simulink library "commdigbbndcpm2"  (Simulink 6.0)
settings: Solver=ode45  SolverMode=SingleTasking  StartTime=0.0  StopTime=10.0  RelTol=1e-3
libraries: commdigbbndcpm2 x6
settings Model: RequirementInfo=9  Creator=tdelve  LastModifiedBy=cvora  ExtModeAutoUpdateStatusClock=off  ProdHWDeviceType=Specified
settings DataIOCC: SignalLoggingName=logsOut
settings OptimizationCC: BooleanDataType=off
settings DebuggingCC: CheckExecutionContextPreStartOutputMsg=on  CheckExecutionContextRuntimeOutputMsg=on  SolverPrmCheckMsg=none
settings HardwareCC: ProdHWDeviceType=Specified
settings SFSimCC: SFSimApplyToAllLibs=on  SFSimBuildMode=Incremental

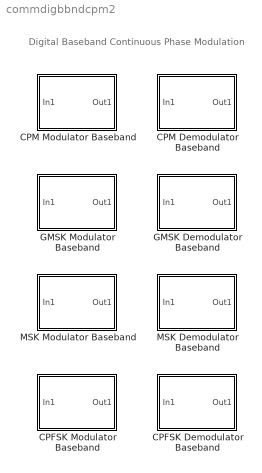
== system commdigbbndcpm2 ==
  note: Digital Baseband
      | Continuous Phase Modulation
  CPFSK Demodulator Baseband : Subsystem  PropExecContextAcrossSSBoundary=on  mask(CPFSK Demodulator Baseband){Mnum=4, outputType=Integer, mappingType=Binary, modIdx=.5, phaseOffset=0, samplesPerSymbol=8, traceBack=16}
      mask prompts: Mnum "M-ary number:"; outputType "Output type:"; mappingType "Symbol set ordering:"; modIdx "Modulation index:"; phaseOffset "Phase offset (rad):"; samplesPerSymbol "Samples per symbol:"; traceBack "Traceback length:"
      mask help:
      | Demodulate the CPFSK modulated input signal using the Viterbi algorithm. Traceback length is the number of trellis branches that the algorithm uses to construct each traceback path.
      |
      | For sample-based input, the input must be a scalar. For frame-based input, the input must be a column vector.
      |
      | The output can be either bits or integers. In case of bit output, the output width is an integer multiple of the number of bits per symbol. The symbols can be either binary-demapped or Gray-demapped into bits.
      |
      | In case of frame-based input, the width of the input frame represents the product of the number of symbols and the Samples per symbol value.
      |
      | In case of sample-based input, the sample time of the input is the symbol period divided by the Samples per symbol value.
      mask init:
      | [eStr,params]=commblkcpfskdemod(gcb, 'init');
      | if(eStr.ecode==1)
      |     error(eStr.emsg);
      | elseif(eStr.ecode==2)
      |     warning(eStr.emsg);
      | end;
      settings: ErrorFcn=commblkcpfskdemod
      mask Help: helpview(commbhelp)
      mask StyleString: edit,popup(Bit|Integer),popup(Binary|Gray),edit,edit,edit,edit
      mask CallbackString: |commblkcpfskdemod(gcb,'cbOutputType');|||||
      mask Display:
      | plot(0,0,100,100,[5+1.5*[[0:.8:10] [10:1.6:20] [20:.8:30]] 50 50 50 50+15*[0 1 1 2 2 3]],[85+10*[sin([0:.8:10]*pi*2/5) sin([10:1.6:20]*pi/5) sin([20:.8:30]*pi*2/5)] 85 99 75 85+8*[1 1 -1 -1 1 1]]);
      | text(50,50,'CPFSK','horiz','center','verti','middle');
  CPFSK Modulator Baseband : Subsystem  PropExecContextAcrossSSBoundary=on  mask(CPFSK Modulator Baseband){Mnum=4, inputType=Integer, mappingType=Binary, modIdx=.5, phaseOffset=0, samplesPerSymbol=8}
      mask prompts: Mnum "M-ary number:"; inputType "Input type:"; mappingType "Symbol set ordering:"; modIdx "Modulation index:"; phaseOffset "Phase offset (rad):"; samplesPerSymbol "Samples per symbol:"
      mask help:
      | Modulate the input signal using the continuous phase frequency shift keying method.
      |
      | The input can be either bits or integers. In case of sample-based bit input, the input width must equal the number of bits per symbol. In case of frame-based bit input, the input width must be an integer multiple of the number of bits per symbol. The bits can be either binary-mapped or Gray-mapped into symbols.
      |
      | For sample-based integer input, the input must be a scalar. For frame-based integer input, the input must be a column vector.
      |
      | In case of frame-based input, the width of the output frame equals the product of the number of symbols and the Samples per symbol value.
      |
      | In case of sample-based input, the output sample time equals the symbol period divided by the Samples per symbol value.
      mask init:
      | [eStr,params]=commblkcpfskmod(gcb, 'init');
      | if(eStr.ecode==1)
      |     error(eStr.emsg);
      | elseif(eStr.ecode==2)
      |     warning(eStr.emsg);
      | end;
      settings: ErrorFcn=commblkcpfskmod
      mask Help: helpview(commbhelp)
      mask StyleString: edit,popup(Bit|Integer),popup(Binary|Gray),edit,edit,edit
      mask CallbackString: |commblkcpfskmod(gcb,'cbInputType');||||
      mask Display:
      | plot(0,0,100,100,[5+15*[0 1 1 2 2 3] 50 50 50 50+1.5*[[0:.8:10] [10:1.6:20] [20:.8:30]]],[85+8*[1 1 -1 -1 1 1] 85 99 75 85+10*[sin([0:.8:10]*pi*2/5) sin([10:1.6:20]*pi/5) sin([20:.8:30]*pi*2/5)]]);
      | text(50,50,'CPFSK','horiz','center','verti','middle');
  CPM Demodulator Baseband : Subsystem  PropExecContextAcrossSSBoundary=on  mask(CPM Demodulator Baseband){Mnum=4, outputType=Integer, mappingType=Binary, modIdx=0.5, pulseShape=Rectangular, BT=0.3, mainLobePulseLength=1, rollOff=0.2, pulseLength=1, preHistory=1, phaseOffset=0, samplesPerSymbol=8, traceBack=16}
      mask prompts: Mnum "M-ary number:"; outputType "Output type:"; mappingType "Symbol set ordering:"; modIdx "Modulation index:"; pulseShape "Frequency pulse shape:"; BT "BT product:"; mainLobePulseLength "Main lobe pulse duration (symbol intervals):"; pulseLength "Pulse length (symbol intervals):"; preHistory "Symbol prehistory:"; phaseOffset "Phase offset (rad):"; samplesPerSymbol "Samples per symbol:"; traceBack "Traceback length:"
      mask help:
      | Demodulate the CPM modulated input signal using the Viterbi algorithm. Traceback length is the number of trellis branches that the algorithm uses to construct each traceback path.
      |
      | For sample-based input, the input must be a scalar. For frame-based input, the input must be a column vector.
      |
      | The output can be either bits or integers. In case of bit output, the output width is an integer multiple of the number of bits per symbol. The symbols can be either binary-demapped or Gray-demapped into bits.
      |
      | In case of frame-based input, the width of the input frame represents the product of the number of symbols and the Samples per symbol value.
      |
      | In case of sample-based input, the sample time of the input is the symbol period divided by the Samples per symbol value.
      mask init:
      | [eStr,params]=commblkcpmdemod(gcb, 'init');
      | if(eStr.ecode==1)
      |     error(eStr.emsg);
      | elseif(eStr.ecode==2)
      |     warning(eStr.emsg);
      | end;
      settings: ErrorFcn=commblkcpmdemod
      mask Help: helpview(commbhelp)
      mask StyleString: edit,popup(Bit|Integer),popup(Binary|Gray),edit,popup(Rectangular|Raised Cosine|Spectral Raised Cosine|Gaussian|Tamed FM),edit,edit,edit,edit,edit,edit,edit,edit
      mask CallbackString: |commblkcpmdemod(gcb,'cbOutputType');|||commblkcpmdemod(gcb,'cbPulseShape');||||||||
      mask Display:
      | plot(0,0,100,100,[5+1.5*[[0:.8:10] [10:1.6:20] [20:.8:30]] 50 50 50 50+15*[0 1 1 2 2 3]],[85+10*[sin([0:.8:10]*pi*2/5) sin([10:1.6:20]*pi/5) sin([20:.8:30]*pi*2/5)] 85 99 75 85+8*[1 1 -1 -1 1 1]]);
      | text(50,50,'CPM','horiz','center','verti','middle');
  CPM Modulator Baseband : Subsystem  PropExecContextAcrossSSBoundary=on  mask(CPM Modulator Baseband){Mnum=4, inputType=Integer, mappingType=Binary, modIdx=0.5, pulseShape=Rectangular, BT=0.3, mainLobePulseLength=1, rollOff=0.2, pulseLength=1, preHistory=1, phaseOffset=0, samplesPerSymbol=8}
      mask prompts: Mnum "M-ary number:"; inputType "Input type:"; mappingType "Symbol set ordering:"; modIdx "Modulation index:"; pulseShape "Frequency pulse shape:"; BT "BT product:"; mainLobePulseLength "Main lobe pulse duration (symbol intervals):"; pulseLength "Pulse length (symbol intervals):"; preHistory "Symbol prehistory:"; phaseOffset "Phase offset (rad):"; samplesPerSymbol "Samples per symbol:"
      mask help:
      | Output the complex envelope representation of the selected continuous phase modulation.
      |
      | The input can be either bits or integers. In case of sample-based bit input, the input width must equal the number of bits per symbol. In case of frame-based bit input, the input width must be an integer multiple of the number of bits per symbol. The bits can be either binary-mapped or Gray-mapped into symbols.
      |
      | For sample-based integer input, the input must be a scalar. For frame-based integer input, the input must be a column vector.
      |
      | In case of frame-based input, the width of the output frame equals the product of the number of symbols and the Samples per symbol value.
      |
      | In case of sample-based input, the output sample time equals the symbol period divided by the Samples per symbol value.
      |
      | The Symbol prehistory parameter is the data symbol(s) used before the start of the simulation.
      mask init:
      | [eStr,params]=commblkcpmmod(gcb, 'init');
      | if(eStr.ecode==1)
      |     error(eStr.emsg);
      | elseif(eStr.ecode==2)
      |     warning(eStr.emsg);
      | end;
      settings: ErrorFcn=commblkcpmmod
      mask Help: helpview(commbhelp)
      mask StyleString: edit,popup(Bit|Integer),popup(Binary|Gray),edit,popup(Rectangular|Raised Cosine|Spectral Raised Cosine|Gaussian|Tamed FM),edit,edit,edit,edit,edit,edit,edit
      mask CallbackString: |commblkcpmmod(gcb,'cbInputType');|||commblkcpmmod(gcb,'cbPulseShape');|||||||
      mask Display:
      | plot(0,0,100,100,[5+15*[0 1 1 2 2 3] 50 50 50 50+1.5*[[0:.8:10] [10:1.6:20] [20:.8:30]]],[85+8*[1 1 -1 -1 1 1] 85 99 75 85+10*[sin([0:.8:10]*pi*2/5) sin([10:1.6:20]*pi/5) sin([20:.8:30]*pi*2/5)]]);
      | text(50,50,'CPM','horiz','center','verti','middle');
  GMSK Demodulator Baseband : Subsystem  PropExecContextAcrossSSBoundary=on  mask(GMSK Demodulator Baseband){OutputType=Integer, BT=.3, pulseLength=4, preHistory=1, phaseOffset=0, samplesPerSymbol=8, traceBack=16}
      mask prompts: OutputType "Output type:"; BT "BT product:"; pulseLength "Pulse length (symbol intervals):"; preHistory "Symbol prehistory:"; phaseOffset "Phase offset (rad):"; samplesPerSymbol "Samples per symbol:"; traceBack "Traceback length:"
      mask help:
      | Demodulate the GMSK modulated input signal using the Viterbi algorithm. Traceback length is the number of trellis branches that the algorithm uses to construct each traceback path.
      |
      | For sample-based input, the input must be a scalar. For frame-based input, the input must be a column vector.
      |
      | In case of frame-based input, the width of the input frame represents the product of the number of symbols and the Samples per symbol value.
      |
      | In case of sample-based input, the sample time of the input is the symbol period divided by the Samples per symbol value.
      |
      | The Symbol prehistory parameter is the data symbol(s) used before the start of the simulation.
      mask init:
      | [eStr,params]=commblkgmskdemod(gcb, 'init');
      | if(eStr.ecode==1)
      |     error(eStr.emsg);
      | elseif(eStr.ecode==2)
      |     warning(eStr.emsg);
      | end;
      settings: ErrorFcn=commblkgmskdemod
      mask Help: helpview(commbhelp)
      mask StyleString: popup(Bit|Integer),edit,edit,edit,edit,edit,edit
      mask Display:
      | plot(0,0,100,100,[5+1.5*[[0:.8:10] [10:1.6:20] [20:.8:30]] 50 50 50 50+15*[0 1 1 2 2 3]],[85+10*[sin([0:.8:10]*pi*2/5) sin([10:1.6:20]*pi/5) sin([20:.8:30]*pi*2/5)] 85 99 75 85+8*[1 1 -1 -1 1 1]]);
      | text(50,50,'GMSK','horiz','center','verti','middle');
  GMSK Modulator Baseband : Subsystem  PropExecContextAcrossSSBoundary=on  mask(GMSK Modulator Baseband){inputType=Integer, BT=.3, pulseLength=4, preHistory=1, phaseOffset=0, samplesPerSymbol=8}
      mask prompts: inputType "Input type:"; BT "BT product:"; pulseLength "Pulse length (symbol intervals):"; preHistory "Symbol prehistory:"; phaseOffset "Phase offset (rad):"; samplesPerSymbol "Samples per symbol:"
      mask help:
      | Modulate the input signal using the Gaussian minimum shift keying method.
      |
      | For sample-based input, the input must be a scalar. For frame-based input, the input must be a column vector.
      |
      | In case of frame-based input, the width of the output frame equals the product of the number of symbols and the Samples per symbol value.
      |
      | In case of sample-based input, the output sample time equals the symbol period divided by the Samples per symbol value.
      |
      | The Symbol prehistory parameter is the data symbol(s) used before the start of the simulation.
      mask init:
      | [eStr,params]=commblkgmskmod(gcb, 'init');
      | if(eStr.ecode==1)
      |     error(eStr.emsg);
      | elseif(eStr.ecode==2)
      |     warning(eStr.emsg);
      | end;
      settings: ErrorFcn=commblkgmskmod
      mask Help: helpview(commbhelp)
      mask StyleString: popup(Bit|Integer),edit,edit,edit,edit,edit
      mask Display:
      | plot(0,0,100,100,[5+15*[0 1 1 2 2 3] 50 50 50 50+1.5*[[0:.8:10] [10:1.6:20] [20:.8:30]]],[85+8*[1 1 -1 -1 1 1] 85 99 75 85+10*[sin([0:.8:10]*pi*2/5) sin([10:1.6:20]*pi/5) sin([20:.8:30]*pi*2/5)]]);
      | text(50,50,'GMSK','horiz','center','verti','middle');
  MSK Demodulator Baseband : Subsystem  PropExecContextAcrossSSBoundary=on  mask(MSK Demodulator Baseband){outputType=Integer, phaseOffset=0, samplesPerSymbol=8, traceBack=16}
      mask prompts: outputType "Output type:"; phaseOffset "Phase offset (rad):"; samplesPerSymbol "Samples per symbol:"; traceBack "Traceback length:"
      mask help:
      | Demodulate the MSK modulated input signal using the Viterbi algorithm. Traceback length is the number of trellis branches that the algorithm uses to construct each traceback path.
      |
      | For sample-based input, the input must be a scalar. For frame-based input, the input must be a column vector.
      |
      | In case of frame-based input, the width of the input frame represents the product of the number of symbols and the Samples per symbol value.
      |
      | In case of sample-based input, the sample time of the input is the symbol period divided by the Samples per symbol value.
      mask init:
      | [eStr,params]=commblkmskdemod(gcb, 'init');
      | if(eStr.ecode==1)
      |     error(eStr.emsg);
      | elseif(eStr.ecode==2)
      |     warning(eStr.emsg);
      | end;
      settings: ErrorFcn=commblkmskdemod
      mask Help: helpview(commbhelp)
      mask StyleString: popup(Bit|Integer),edit,edit,edit
      mask Display:
      | plot(0,0,100,100,[5+1.5*[[0:.8:10] [10:1.6:20] [20:.8:30]] 50 50 50 50+15*[0 1 1 2 2 3]],[85+10*[sin([0:.8:10]*pi*2/5) sin([10:1.6:20]*pi/5) sin([20:.8:30]*pi*2/5)] 85 99 75 85+8*[1 1 -1 -1 1 1]]);
      | text(51,51,'MSK','horiz','center','verti','middle');
  MSK Modulator Baseband : Subsystem  PropExecContextAcrossSSBoundary=on  mask(MSK Modulator Baseband){inputType=Integer, phaseOffset=0, samplesPerSymbol=8}
      mask prompts: inputType "Input type:"; phaseOffset "Phase offset (rad):"; samplesPerSymbol "Samples per symbol:"
      mask help:
      | Modulate the input signal using the minimum shift keying method.
      |
      | For sample-based input, the input must be a scalar. For frame-based input, the input must be a column vector.
      |
      | In case of frame-based input, the width of the output frame equals the product of the number of symbols and the Samples per symbol value.
      |
      | In case of sample-based input, the output sample time equals the symbol period divided by the Samples per symbol value.
      mask init:
      | [eStr,params]=commblkmskmod(gcb, 'init');
      | if(eStr.ecode==1)
      |     error(eStr.emsg);
      | elseif(eStr.ecode==2)
      |     warning(eStr.emsg);
      | end;
      settings: ErrorFcn=commblkmskmod
      mask Help: helpview(commbhelp)
      mask StyleString: popup(Bit|Integer),edit,edit
      mask Display:
      | plot(0,0,100,100,[5+15*[0 1 1 2 2 3] 50 50 50 50+1.5*[[0:.8:10] [10:1.6:20] [20:.8:30]]],[85+8*[1 1 -1 -1 1 1] 85 99 75 85+10*[sin([0:.8:10]*pi*2/5) sin([10:1.6:20]*pi/5) sin([20:.8:30]*pi*2/5)]]);
      | text(51,51,'MSK','horiz','center','verti','middle');

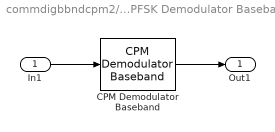
== system commdigbbndcpm2/CPFSK Demodulator Baseband ==
  In1 : Inport  LatchInput=off
  CPM Demodulator Baseband : commdigbbndcpm2/CPM Demodulator Baseband  Mnum=Mnum  outputType=Integer  mappingType=Binary  modIdx=modIdx  pulseShape=Rectangular  BT=.3  mainLobePulseLength=1  rollOff=0.2  pulseLength=1  preHistory=1  phaseOffset=phaseOffset  samplesPerSymbol=samplesPerSymbol  traceBack=traceBack
  Out1 : Outport
  wires:
  CPM Demodulator Baseband/1 -> Out1/1
  In1/1 -> CPM Demodulator Baseband/1

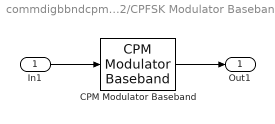
== system commdigbbndcpm2/CPFSK Modulator Baseband ==
  In1 : Inport  LatchInput=off
  CPM Modulator Baseband : commdigbbndcpm2/CPM Modulator Baseband  Mnum=Mnum  inputType=Integer  mappingType=Binary  modIdx=modIdx  pulseShape=Rectangular  BT=0.3  mainLobePulseLength=0.2  rollOff=0.2  pulseLength=1  preHistory=1  phaseOffset=0  samplesPerSymbol=samplesPerSymbol
  Out1 : Outport
  wires:
  In1/1 -> CPM Modulator Baseband/1
  CPM Modulator Baseband/1 -> Out1/1

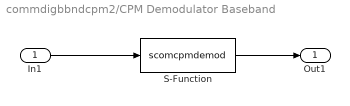
== system commdigbbndcpm2/CPM Demodulator Baseband ==
  In1 : Inport  LatchInput=off
  S-Function : S-Function  FunctionName=scomcpmdemod  Parameters=Mnum,outputType,mappingType,modIdx,pulseShape,BT,mainLobePulseLength,rollOff,pulseLength,phaseOffset,samplesPerSymbol, params.gMod,preHistory,0,traceBack,params.m,params.p  SFunctionModules=buff cpmmodulation trellisdecode phasetrellis
  Out1 : Outport
  wires:
  S-Function/1 -> Out1/1
  In1/1 -> S-Function/1

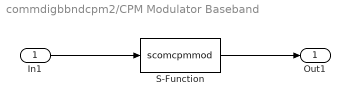
== system commdigbbndcpm2/CPM Modulator Baseband ==
  In1 : Inport  LatchInput=off
  S-Function : S-Function  FunctionName=scomcpmmod  Parameters=Mnum,inputType,mappingType,modIdx,pulseShape,BT,mainLobePulseLength,rollOff,pulseLength,phaseOffset,samplesPerSymbol, params.gMod,preHistory,0  SFunctionModules=buff cpmmodulation
  Out1 : Outport
  wires:
  In1/1 -> S-Function/1
  S-Function/1 -> Out1/1

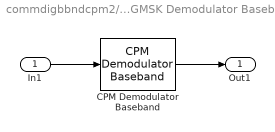
== system commdigbbndcpm2/GMSK Demodulator Baseband ==
  In1 : Inport  LatchInput=off
  CPM Demodulator Baseband : commdigbbndcpm2/CPM Demodulator Baseband  Mnum=2  outputType=Integer  mappingType=Binary  modIdx=0.5  pulseShape=Gaussian  BT=BT  mainLobePulseLength=1  rollOff=0.2  pulseLength=pulseLength  preHistory=preHistory  phaseOffset=phaseOffset  samplesPerSymbol=samplesPerSymbol  traceBack=traceBack
  Out1 : Outport
  wires:
  CPM Demodulator Baseband/1 -> Out1/1
  In1/1 -> CPM Demodulator Baseband/1

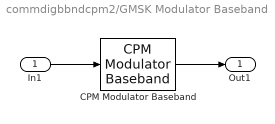
== system commdigbbndcpm2/GMSK Modulator Baseband ==
  In1 : Inport  LatchInput=off
  CPM Modulator Baseband : commdigbbndcpm2/CPM Modulator Baseband  Mnum=2  inputType=Integer  mappingType=Binary  modIdx=.5  pulseShape=Gaussian  BT=BT  mainLobePulseLength=0.2  rollOff=0.2  pulseLength=pulseLength  preHistory=preHistory  phaseOffset=phaseOffset  samplesPerSymbol=samplesPerSymbol
  Out1 : Outport
  wires:
  In1/1 -> CPM Modulator Baseband/1
  CPM Modulator Baseband/1 -> Out1/1

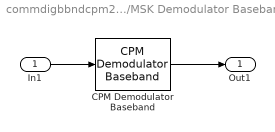
== system commdigbbndcpm2/MSK Demodulator Baseband ==
  In1 : Inport  LatchInput=off
  CPM Demodulator Baseband : commdigbbndcpm2/CPM Demodulator Baseband  Mnum=2  outputType=Integer  mappingType=Binary  modIdx=0.5  pulseShape=Rectangular  BT=.3  mainLobePulseLength=1  rollOff=0.2  pulseLength=1  preHistory=1  phaseOffset=phaseOffset  samplesPerSymbol=samplesPerSymbol  traceBack=traceBack
  Out1 : Outport
  wires:
  CPM Demodulator Baseband/1 -> Out1/1
  In1/1 -> CPM Demodulator Baseband/1

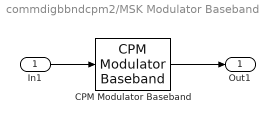
== system commdigbbndcpm2/MSK Modulator Baseband ==
  In1 : Inport  LatchInput=off
  CPM Modulator Baseband : commdigbbndcpm2/CPM Modulator Baseband  Mnum=2  inputType=Integer  mappingType=Binary  modIdx=0.5  pulseShape=Rectangular  BT=0.3  mainLobePulseLength=0.2  rollOff=0.2  pulseLength=1  preHistory=1  phaseOffset=phaseOffset  samplesPerSymbol=samplesPerSymbol
  Out1 : Outport
  wires:
  In1/1 -> CPM Modulator Baseband/1
  CPM Modulator Baseband/1 -> Out1/1
